simulink subsystem "flight_path"  (R2020a)
settings: Solver=VariableStepAuto  StartTime=0.0  StopTime=10.0  RelTol=1e-3
values from neighbouring files (symbols this model uses):
  dt = 0.01    [configure_simulation.m]    (also in test_kalman.m)
  initial_latitude = 39.5296    [configure_simulation.m]
  initial_longitude = -119.8138    [configure_simulation.m]
undefined symbols (not defined in the file or in its folder): Earth, WGS84
libraries: aerolibtransform2 x2
settings Model: Creator=Philip  LastModifiedBy=Philip

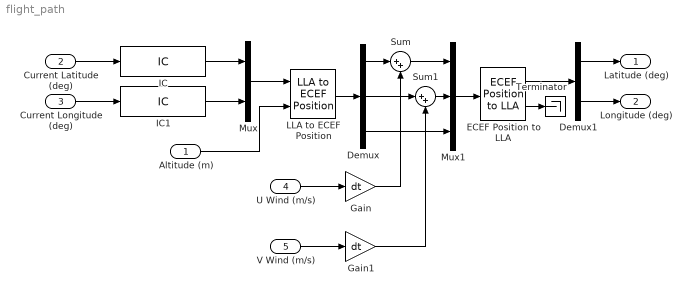
== system flight_path ==
  Altitude (m) : Inport
  Current Latitude (deg) : Inport  Port=2
  Current Longitude (deg) : Inport  Port=3
  U Wind (m/s) : Inport  Port=4
  V Wind (m/s) : Inport  Port=5
  Demux : Demux  Outputs=3
  Demux1 : Demux  Outputs=2
  ECEF Position to LLA : aerolibtransform2/ECEF Position to LLA  units=Metric (MKS)  ptype=Earth (WGS84)  F=1/298.257223563  R=6378137
      settings: SourceProductBaseCode=AE
  Gain : Gain  Gain=dt
  Gain1 : Gain  Gain=dt
  IC : InitialCondition  Value=initial_latitude
  IC1 : InitialCondition  Value=initial_longitude
  LLA to ECEF Position : aerolibtransform2/LLA to ECEF Position  units=Metric (MKS)  ptype=Earth (WGS84)  F=1/298.257223563  R=6378137
      settings: SourceProductBaseCode=AE
  Mux : Mux  Inputs=2
  Mux1 : Mux  Inputs=3
  Sum : Sum  Inputs=|++
  Sum1 : Sum  Inputs=|++
  Terminator : Terminator
  Latitude (deg) : Outport
  Longitude (deg) : Outport  Port=2
  wires:
  Demux1/1 -> Latitude (deg)/1
  Demux1/2 -> Longitude (deg)/1
  Gain1/1 -> Sum1/2
  U Wind (m/s)/1 -> Gain/1
  V Wind (m/s)/1 -> Gain1/1
  Gain/1 -> Sum/2
  Current Latitude (deg)/1 -> IC/1
  Current Longitude (deg)/1 -> IC1/1
  Mux/1 -> LLA to ECEF Position/1
  Altitude (m)/1 -> LLA to ECEF Position/2
  ECEF Position to LLA/2 -> Terminator/1
  LLA to ECEF Position/1 -> Demux/1
  Demux/1 -> Sum/1
  Demux/2 -> Sum1/1
  Sum1/1 -> Mux1/2
  Sum/1 -> Mux1/1
  Demux/3 -> Mux1/3
  Mux1/1 -> ECEF Position to LLA/1
  ECEF Position to LLA/1 -> Demux1/1
  IC/1 -> Mux/1
  IC1/1 -> Mux/2
